simulink model "dart_AUV_simulink_model"  (R2024b)
settings: Solver=VariableStepAuto  StartTime=0.0  StopTime=20  RelTol=1e-3
values from neighbouring files (symbols this model uses):
  Af = [0.5; 0.1; 0.5]    [init_param.m]
  Bc = [0, 0, 0.042]    [init_param.m]
  Cg = [0, 0, 0.021]    [init_param.m]
  Delta_2 = Delta.^2    [init_param.m]
  DL = diag([Xu, 0, 0, 0, 0, 0 ... (first row only)    [init_param.m]
  DNL = diag([Xu_nl, 0, 0, 0, 0, 0 ... (first row only)    [init_param.m]
  I = [Ixx,Iyy, Izz, Ixy, Ixz, Iyz]    [init_param.m]
  L = 0.47    [init_param.m]
  m = 2.24    [init_param.m]
  Ma = [ ... (first row only)    [init_param.m]
  Mt = Mb + Ma    [init_param.m]
  Omega = [0.085; 0.085; 0.9]    [init_param.m]
  R = d / 2    (= 0.04445)    [init_param.m]
  rho = 1025    [init_param.m]
undefined symbols (not defined in the file or in its folder): CD, CL, fractalcoef
libraries: slpidlib x3, mspfiltlib x1, mspsensorlib x1, mpclib x1
settings Model: Creator=tihan  LastModifiedBy=tihan

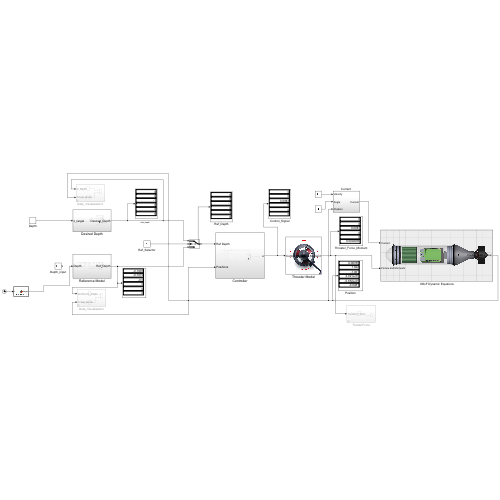
[thumbnail: Simulink's stored preview of the top-level diagram]
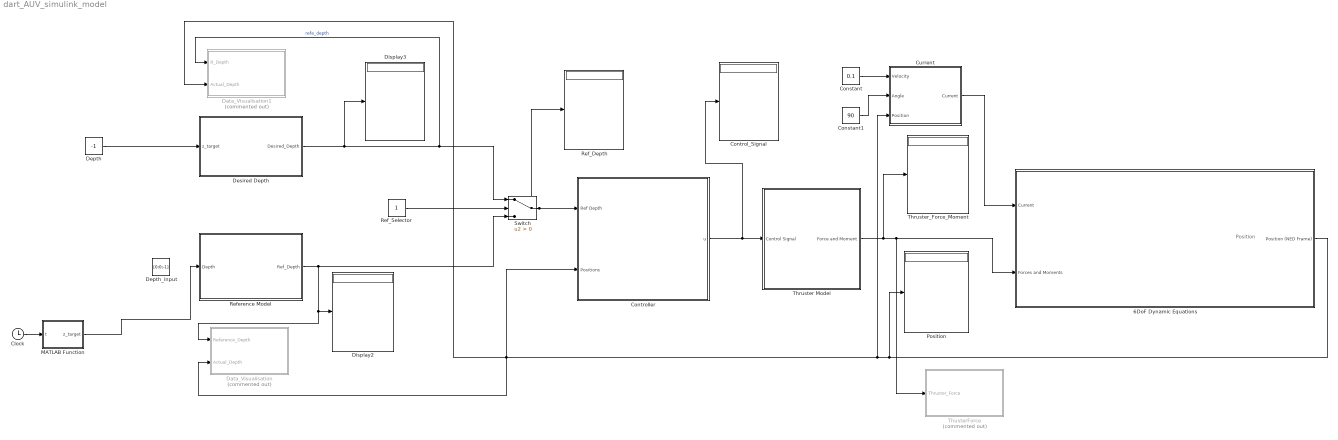
== system dart_AUV_simulink_model ==
  note: Position
  " 6DoF Dynamic Equations " : Subsystem
      mask Display: image('image.png');
  Clock : Clock
  Constant : Constant  Value=0.1
  Constant1 : Constant  Value=90
  Control_Signal : Display
  Controller : Subsystem
  "Current " : Subsystem
  Data_Visualisation : Subsystem  Commented=on
  Data_Visualisation1 : Subsystem  Commented=on
  Depth : Constant  Value=-1
  Depth_input : Constant  Value=[0;0;-1]
  Desired Depth : Subsystem
  Display2 : Display
  Display3 : Display
  MATLAB Function : MATLAB Function  TreatAsAtomicUnit=on
  Position : Display
  Ref_Depth : Display
  Ref_Selector : Constant
  Reference Model : Subsystem
  Switch : Switch  Criteria=u2 > Threshold  SaturateOnIntegerOverflow=off  InputSameDT=off
  Thruster Model : Subsystem
      mask Display: image('thruster_small.jpg');
  Thruster_Force_Moment : Display
  ThusterForce : Subsystem  Commented=on
  wires:
  Controller/1(u) -> Thruster Model/1(Control Signal), Control_Signal/1
  " 6DoF Dynamic Equations "/1(Position (NED Frame)) -> Position/1, Controller/2(Positions), Data_Visualisation1/2(Actual_Depth), Data_Visualisation/2(Actual_Depth), "Current "/3(Position)
  Thruster Model/1(Force and Moment) -> ThusterForce/1(Thruster_Force), " 6DoF Dynamic Equations "/2("Forces and Moments  "), Thruster_Force_Moment/1
  Reference Model/1(Ref_Depth) -> Switch/3, Data_Visualisation/1(Reference_Depth), Display2/1
  "Current "/1(Current) -> " 6DoF Dynamic Equations "/1(Current)
  Constant/1 -> "Current "/1(Velocity)
  Constant1/1 -> "Current "/2(Angle)
  Ref_Selector/1 -> Switch/2
  Switch/1 -> Controller/1(Ref Depth), Ref_Depth/1
  Desired Depth/1(Desired_Depth) -> Display3/1, Data_Visualisation1/1(R_Depth), Switch/1  "refe_depth"
  Clock/1 -> MATLAB Function/1(t)
  MATLAB Function/1(z_target) -> Reference Model/1(Depth)
  Depth/1 -> Desired Depth/1(z_target)

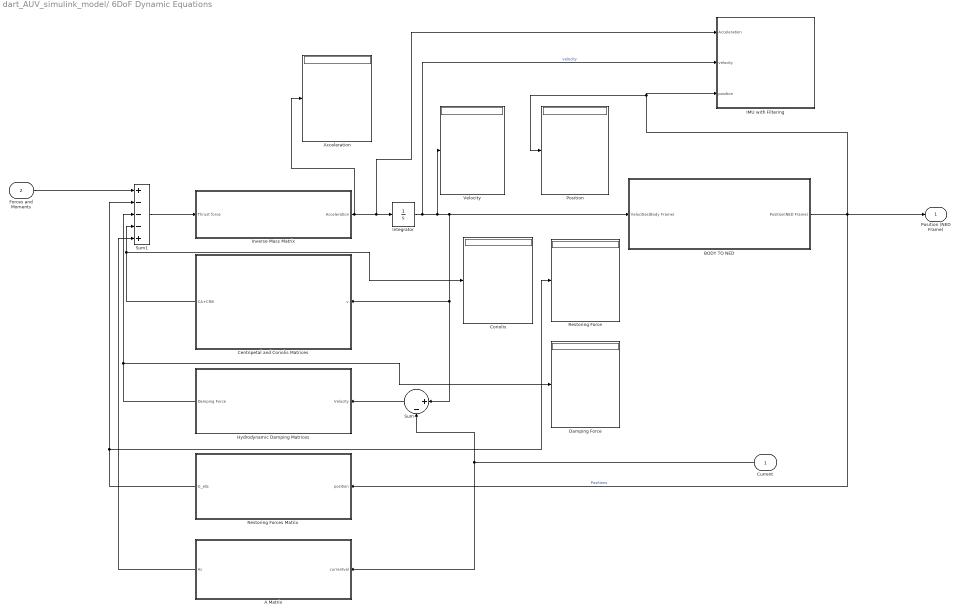
== system dart_AUV_simulink_model/ 6DoF Dynamic Equations  ==
  Current : Inport
  "Forces and Moments  " : Inport  Port=2
  " A Matrix" : Subsystem
  Acceleration : Display
  BODY TO NED : Subsystem
  "Centripetal and Coriolis Matrices " : Subsystem
  Coriolis : Display
  Damping Force : Display
  "Hydrodynamic Damping Matrices " : Subsystem
  IMU with Filtering : Subsystem
  Integrator : Integrator
  Inverse Mass Matrix : Subsystem
  Position : Display
  Restoring Force : Display
  Restoring Forces Matrix : Subsystem
  Sum : Sum  Inputs=|+-
  Sum1 : Sum  Inputs=+---+  InputSameDT=on  SaturateOnIntegerOverflow=on  OutDataTypeStr=Inherit: Same as first input
  Velocity : Display
  Position (NED Frame) : Outport  VectorParamsAs1DForOutWhenUnconnected=off
  wires:
  Restoring Forces Matrix/1(G_eta) -> Restoring Force/1, Sum1/2
  Sum1/1 -> Inverse Mass Matrix/1(Thrust force)
  "Forces and Moments  "/1 -> Sum1/1
  "Centripetal and Coriolis Matrices "/1(CA+CRB) -> Coriolis/1, Sum1/4
  Sum/1 -> "Hydrodynamic Damping Matrices "/1(Velocity)
  Current/1 -> " A Matrix"/1(currentvel), Sum/2
  " A Matrix"/1(Ac) -> Sum1/5
  Inverse Mass Matrix/1(Acceleration) -> IMU with Filtering/1(Acceleration), Integrator/1, Acceleration/1
  Integrator/1 -> IMU with Filtering/2(velocity), Velocity/1, "Centripetal and Coriolis Matrices "/1(v), Sum/1, BODY TO NED/1(Velocities(Body Frame))  "velocity"
  "Hydrodynamic Damping Matrices "/1(Damping Force) -> Damping Force/1, Sum1/3
  BODY TO NED/1(" Position(NED Frame)") -> Restoring Forces Matrix/1(position), IMU with Filtering/3(position), Position/1, Position (NED Frame)/1  "Positions"

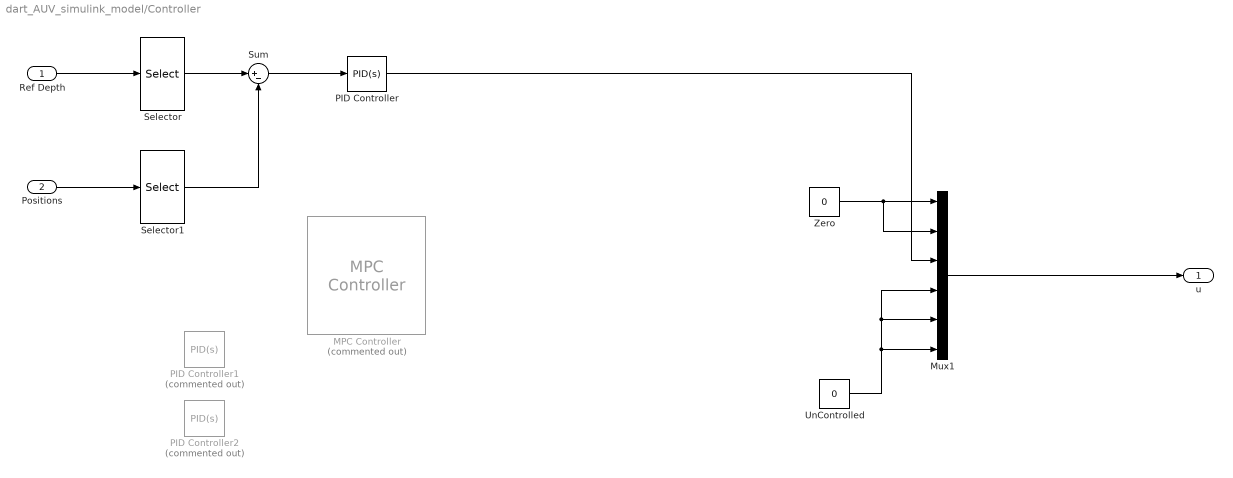
== system dart_AUV_simulink_model/Controller ==
  Ref Depth : Inport
  Positions : Inport  Port=2
  MPC Controller : mpclib/MPC Controller  Commented=on  SCDEnableBlockLinearizationSpecification=on  is_multiple=0  enable_value=0  return_u0=off  updateMPCinCallerWorkspace=on  md_inport=off  mv_inport=off  uref_inport=off  return_cost=off  return_mvseq=off  return_qpstatus=off  return_xseq=off  return_state=off  return_ovseq=off  state_inport=off  umin_inport=off  umax_inport=off  ymin_inport=off  ymax_inport=off  cc_inport=off  ywt_inport=off  uwt_inport=off  duwt_inport=off  rhoeps_inport=off  pm_inport=off  MaximumP=10  HorizonChoice=FixedHorizon  n_ts=1  n_p=10  n_mv=1  n_md=1  n_ud=0  n_mo=1  n_uo=0  BlockDataType=double  SampleTimeInherited=off  switch_inport=off
  Mux1 : Mux  Inputs=6
  PID Controller : slpidlib/PID Controller  Controller=PID  Form=Parallel  TimeDomain=Continuous-time  UseExternalTs=off  SampleTime=-1  IntegratorMethod=Forward Euler  FilterMethod=Forward Euler  ControllerParametersSource=internal  P=80  I=0.001  UseKiTs=off  D=50  UseExternalDerivativeSource=off  N=114.923982318212  UseFilter=on  TunerSelectOption=Transfer Function Based (PID Tuner App)  InitialConditionSource=internal  InitialConditionForIntegrator=0  InitialConditionForFilter=0  DifferentiatorICPrevScaledInput=0  ExternalReset=none  TrackingMode=off  Kt=1  LimitOutput=off  SatLimitsSource=internal  UpperSaturationLimit=inf  LowerSaturationLimit=-inf  LinearizeAsGain=on  AntiWindupMode=none  Kb=1  LimitIntegrator=off  UpperIntegratorSaturationLimit=inf  LowerIntegratorSaturationLimit=-inf  POutMin=[]  POutMax=[]  IOutMin=[]  IOutMax=[]  DOutMin=[]  DOutMax=[]  NOutMin=[]  NOutMax=[]  SumOutMin=[]  SumOutMax=[]  SaturationOutMin=[]  SaturationOutMax=[]  PParamMin=[]  PParamMax=[]  IParamMin=[]  IParamMax=[]  DParamMin=[]  DParamMax=[]  NParamMin=[]  NParamMax=[]  KbParamMin=[]  KbParamMax=[]  KtParamMin=[]  KtParamMax=[]  KbOutMin=[]  KbOutMax=[]  KtOutMin=[]  KtOutMax=[]  IntegratorOutMin=[]  IntegratorOutMax=[]  FilterOutMin=[]  FilterOutMax=[]  SumI1OutMin=[]  SumI1OutMax=[]  SumI2OutMin=[]  SumI2OutMax=[]  SumI3OutMin=[]  SumI3OutMax=[]  SumI4OutMin=[]  SumI4OutMax=[]  SumDOutMin=[]  SumDOutMax=[]  DifferentiatorOutMin=[]  DifferentiatorOutMax=[]  FilterDiffOutCoefMin=[]  FilterDiffOutCoefMax=[]  ReciprocalOutMin=[]  ReciprocalOutMax=[]  SumDenOutMin=[]  SumDenOutMax=[]  SumNumOutMin=[]  SumNumOutMax=[]  DivideOutMin=[]  DivideOutMax=[]  UdiffTsProdOutMin=[]  UdiffTsProdOutMax=[]  NTsProdOutMin=[]  NTsProdOutMax=[]  UintegralTsProdOutMin=[]  UintegralTsProdOutMax=[]  UngainTsProdOutMin=[]  UngainTsProdOutMax=[]  ClampingZeroOutDataTypeStr=Inherit: Inherit via back propagation  ClampingZeroOutMin=[]  ClampingZeroOutMax=[]  FilterDenConstantOutDataTypeStr=Inherit: Inherit via back propagation  FilterDenConstantOutMin=[]  FilterDenConstantOutMax=[]  PCopyOutDataTypeStr=Inherit: Inherit via back propagation  PCopyOutMin=[]  PCopyOutMax=[]  NCopyOutDataTypeStr=Inherit: Inherit via back propagation  NCopyOutMin=[]  NCopyOutMax=[]  IntegratorContinuousStateAttributes=''  IntegratorStateMustResolveToSignalObject=off  IntegratorRTWStateStorageClass=Auto  FilterContinuousStateAttributes=''  FilterStateMustResolveToSignalObject=off  FilterRTWStateStorageClass=Auto  ParallelPVariant=InternalParameters  IdealPVariant=Disabled  IVariant=InternalParameters  DVariant=InternalParameters  IntegratorVariant=Continuous  SatVariant=Disabled  AWVariant=Passthrough  PCopyVariant=Disabled  TRVariant=Disabled  FdbkBlocksVariant=Forward  IdealPFdbkVariant=Disabled  SatFdbkVariant=Disabled  DerivativeFilterVariant=ContFilter  NVariant=InternalParameters  NCopyVariant=Disabled  FilterICVariant=InternalICsFilter  IntegratorICVariant=InternalICs  ExternalResetVariant=Disabled  TRSumVariant=Passthrough  SumFdbkVariant=Disabled  SumVariant=Sum_PID  TsampFilterVariant=InternalTs  TsampNgainVariant=Passthrough  TsampIntegralVariant=Disabled_SignalSpec  ExternalSaturationOutDataTypeStr=Inherit: Same as second input  DerivativeSourceVariant=ErrorSignal  PreIntVariant=InternalPreInt
  PID Controller1 : slpidlib/PID Controller  Commented=on  Controller=PID  Form=Parallel  TimeDomain=Continuous-time  UseExternalTs=off  SampleTime=-1  IntegratorMethod=Forward Euler  FilterMethod=Forward Euler  ControllerParametersSource=internal  P=90  I=0.1  UseKiTs=off  D=70  UseExternalDerivativeSource=off  N=257.686519224459  UseFilter=on  TunerSelectOption=Transfer Function Based (PID Tuner App)  InitialConditionSource=internal  InitialConditionForIntegrator=0  InitialConditionForFilter=0  DifferentiatorICPrevScaledInput=0  ExternalReset=none  TrackingMode=off  Kt=1  LimitOutput=off  SatLimitsSource=internal  UpperSaturationLimit=inf  LowerSaturationLimit=-inf  LinearizeAsGain=on  AntiWindupMode=none  Kb=1  LimitIntegrator=off  UpperIntegratorSaturationLimit=inf  LowerIntegratorSaturationLimit=-inf  POutMin=[]  POutMax=[]  IOutMin=[]  IOutMax=[]  DOutMin=[]  DOutMax=[]  NOutMin=[]  NOutMax=[]  SumOutMin=[]  SumOutMax=[]  SaturationOutMin=[]  SaturationOutMax=[]  PParamMin=[]  PParamMax=[]  IParamMin=[]  IParamMax=[]  DParamMin=[]  DParamMax=[]  NParamMin=[]  NParamMax=[]  KbParamMin=[]  KbParamMax=[]  KtParamMin=[]  KtParamMax=[]  KbOutMin=[]  KbOutMax=[]  KtOutMin=[]  KtOutMax=[]  IntegratorOutMin=[]  IntegratorOutMax=[]  FilterOutMin=[]  FilterOutMax=[]  SumI1OutMin=[]  SumI1OutMax=[]  SumI2OutMin=[]  SumI2OutMax=[]  SumI3OutMin=[]  SumI3OutMax=[]  SumI4OutMin=[]  SumI4OutMax=[]  SumDOutMin=[]  SumDOutMax=[]  DifferentiatorOutMin=[]  DifferentiatorOutMax=[]  FilterDiffOutCoefMin=[]  FilterDiffOutCoefMax=[]  ReciprocalOutMin=[]  ReciprocalOutMax=[]  SumDenOutMin=[]  SumDenOutMax=[]  SumNumOutMin=[]  SumNumOutMax=[]  DivideOutMin=[]  DivideOutMax=[]  UdiffTsProdOutMin=[]  UdiffTsProdOutMax=[]  NTsProdOutMin=[]  NTsProdOutMax=[]  UintegralTsProdOutMin=[]  UintegralTsProdOutMax=[]  UngainTsProdOutMin=[]  UngainTsProdOutMax=[]  ClampingZeroOutDataTypeStr=Inherit: Inherit via back propagation  ClampingZeroOutMin=[]  ClampingZeroOutMax=[]  FilterDenConstantOutDataTypeStr=Inherit: Inherit via back propagation  FilterDenConstantOutMin=[]  FilterDenConstantOutMax=[]  PCopyOutDataTypeStr=Inherit: Inherit via back propagation  PCopyOutMin=[]  PCopyOutMax=[]  NCopyOutDataTypeStr=Inherit: Inherit via back propagation  NCopyOutMin=[]  NCopyOutMax=[]  IntegratorContinuousStateAttributes=''  IntegratorStateMustResolveToSignalObject=off  IntegratorRTWStateStorageClass=Auto  FilterContinuousStateAttributes=''  FilterStateMustResolveToSignalObject=off  FilterRTWStateStorageClass=Auto  ParallelPVariant=InternalParameters  IdealPVariant=Disabled  IVariant=InternalParameters  DVariant=InternalParameters  IntegratorVariant=Continuous  SatVariant=Disabled  AWVariant=Passthrough  PCopyVariant=Disabled  TRVariant=Disabled  FdbkBlocksVariant=Forward  IdealPFdbkVariant=Disabled  SatFdbkVariant=Disabled  DerivativeFilterVariant=ContFilter  NVariant=InternalParameters  NCopyVariant=Disabled  FilterICVariant=InternalICsFilter  IntegratorICVariant=InternalICs  ExternalResetVariant=Disabled  TRSumVariant=Passthrough  SumFdbkVariant=Disabled  SumVariant=Sum_PID  TsampFilterVariant=InternalTs  TsampNgainVariant=Passthrough  TsampIntegralVariant=Disabled_SignalSpec  ExternalSaturationOutDataTypeStr=Inherit: Same as second input  DerivativeSourceVariant=ErrorSignal  PreIntVariant=InternalPreInt
  PID Controller2 : slpidlib/PID Controller  Commented=on  Controller=PID  Form=Parallel  TimeDomain=Continuous-time  UseExternalTs=off  SampleTime=-1  IntegratorMethod=Forward Euler  FilterMethod=Forward Euler  ControllerParametersSource=internal  P=90  I=.1  UseKiTs=off  D=70  UseExternalDerivativeSource=off  N=257.686519224459  UseFilter=on  TunerSelectOption=Transfer Function Based (PID Tuner App)  InitialConditionSource=internal  InitialConditionForIntegrator=0  InitialConditionForFilter=0  DifferentiatorICPrevScaledInput=0  ExternalReset=none  TrackingMode=off  Kt=1  LimitOutput=off  SatLimitsSource=internal  UpperSaturationLimit=inf  LowerSaturationLimit=-inf  LinearizeAsGain=on  AntiWindupMode=none  Kb=1  LimitIntegrator=off  UpperIntegratorSaturationLimit=inf  LowerIntegratorSaturationLimit=-inf  POutMin=[]  POutMax=[]  IOutMin=[]  IOutMax=[]  DOutMin=[]  DOutMax=[]  NOutMin=[]  NOutMax=[]  SumOutMin=[]  SumOutMax=[]  SaturationOutMin=[]  SaturationOutMax=[]  PParamMin=[]  PParamMax=[]  IParamMin=[]  IParamMax=[]  DParamMin=[]  DParamMax=[]  NParamMin=[]  NParamMax=[]  KbParamMin=[]  KbParamMax=[]  KtParamMin=[]  KtParamMax=[]  KbOutMin=[]  KbOutMax=[]  KtOutMin=[]  KtOutMax=[]  IntegratorOutMin=[]  IntegratorOutMax=[]  FilterOutMin=[]  FilterOutMax=[]  SumI1OutMin=[]  SumI1OutMax=[]  SumI2OutMin=[]  SumI2OutMax=[]  SumI3OutMin=[]  SumI3OutMax=[]  SumI4OutMin=[]  SumI4OutMax=[]  SumDOutMin=[]  SumDOutMax=[]  DifferentiatorOutMin=[]  DifferentiatorOutMax=[]  FilterDiffOutCoefMin=[]  FilterDiffOutCoefMax=[]  ReciprocalOutMin=[]  ReciprocalOutMax=[]  SumDenOutMin=[]  SumDenOutMax=[]  SumNumOutMin=[]  SumNumOutMax=[]  DivideOutMin=[]  DivideOutMax=[]  UdiffTsProdOutMin=[]  UdiffTsProdOutMax=[]  NTsProdOutMin=[]  NTsProdOutMax=[]  UintegralTsProdOutMin=[]  UintegralTsProdOutMax=[]  UngainTsProdOutMin=[]  UngainTsProdOutMax=[]  ClampingZeroOutDataTypeStr=Inherit: Inherit via back propagation  ClampingZeroOutMin=[]  ClampingZeroOutMax=[]  FilterDenConstantOutDataTypeStr=Inherit: Inherit via back propagation  FilterDenConstantOutMin=[]  FilterDenConstantOutMax=[]  PCopyOutDataTypeStr=Inherit: Inherit via back propagation  PCopyOutMin=[]  PCopyOutMax=[]  NCopyOutDataTypeStr=Inherit: Inherit via back propagation  NCopyOutMin=[]  NCopyOutMax=[]  IntegratorContinuousStateAttributes=''  IntegratorStateMustResolveToSignalObject=off  IntegratorRTWStateStorageClass=Auto  FilterContinuousStateAttributes=''  FilterStateMustResolveToSignalObject=off  FilterRTWStateStorageClass=Auto  ParallelPVariant=InternalParameters  IdealPVariant=Disabled  IVariant=InternalParameters  DVariant=InternalParameters  IntegratorVariant=Continuous  SatVariant=Disabled  AWVariant=Passthrough  PCopyVariant=Disabled  TRVariant=Disabled  FdbkBlocksVariant=Forward  IdealPFdbkVariant=Disabled  SatFdbkVariant=Disabled  DerivativeFilterVariant=ContFilter  NVariant=InternalParameters  NCopyVariant=Disabled  FilterICVariant=InternalICsFilter  IntegratorICVariant=InternalICs  ExternalResetVariant=Disabled  TRSumVariant=Passthrough  SumFdbkVariant=Disabled  SumVariant=Sum_PID  TsampFilterVariant=InternalTs  TsampNgainVariant=Passthrough  TsampIntegralVariant=Disabled_SignalSpec  ExternalSaturationOutDataTypeStr=Inherit: Same as second input  DerivativeSourceVariant=ErrorSignal  PreIntVariant=InternalPreInt
  Selector : Selector  InputPortWidth=6  IndexOptions=Index vector (dialog)  Indices=[3]  OutputSizes=1
  Selector1 : Selector  InputPortWidth=6  IndexOptions=Index vector (dialog)  Indices=[3]  OutputSizes=1
  Sum : Sum  Inputs=|+-
  UnControlled : Constant  Value=0
  Zero : Constant  Value=0
  u : Outport
  wires:
  Ref Depth/1 -> Selector/1
  Positions/1 -> Selector1/1
  Selector/1 -> Sum/1
  Selector1/1 -> Sum/2
  Sum/1 -> PID Controller/1
  Zero/1 -> Mux1/2, Mux1/1
  Mux1/1 -> u/1
  UnControlled/1 -> Mux1/4, Mux1/5, Mux1/6
  PID Controller/1 -> Mux1/3

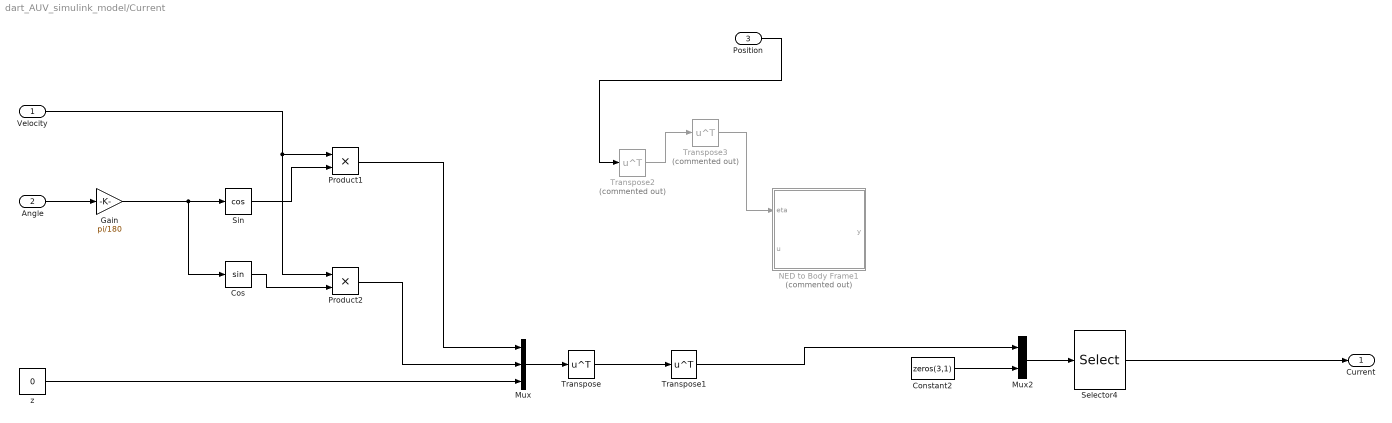
== system dart_AUV_simulink_model/Current  ==
  Velocity : Inport
  Angle : Inport  Port=2
  Position : Inport  Port=3
  Constant2 : Constant  Value=zeros(3,1)
  Cos : Trigonometry
  Gain : Gain  Gain=pi/180
  Mux : Mux  Inputs=3
  Mux2 : Mux  Inputs=2
  NED to Body Frame1 : MATLAB Function  Commented=on  TreatAsAtomicUnit=on
  Product1 : Product
  Product2 : Product
  Selector4 : Selector  InputPortWidth=6  IndexOptions=Index vector (dialog)  Indices=[1 2 4 5 6 3]  OutputSizes=1
  Sin : Trigonometry  Operator=cos  OutputSignalType=real
  Transpose : Math  Operator=transpose
  Transpose1 : Math  Operator=transpose
  Transpose2 : Math  Commented=on  Operator=transpose
  Transpose3 : Math  Commented=on  Operator=transpose
  z : Constant  Value=0
  Current : Outport  VectorParamsAs1DForOutWhenUnconnected=off
  wires:
  Selector4/1 -> Current/1
  Mux2/1 -> Selector4/1
  Mux/1 -> Transpose/1
  Velocity/1 -> Product2/1, Product1/1
  Sin/1 -> Product1/2
  Cos/1 -> Product2/2
  Product1/1 -> Mux/1
  Product2/1 -> Mux/2
  z/1 -> Mux/3
  Transpose/1 -> Transpose1/1
  Angle/1 -> Gain/1
  Constant2/1 -> Mux2/2
  Gain/1 -> Cos/1, Sin/1
  Transpose2/1 -> Transpose3/1
  Transpose3/1 -> NED to Body Frame1/1(eta)
  Position/1 -> Transpose2/1
  Transpose1/1 -> Mux2/1

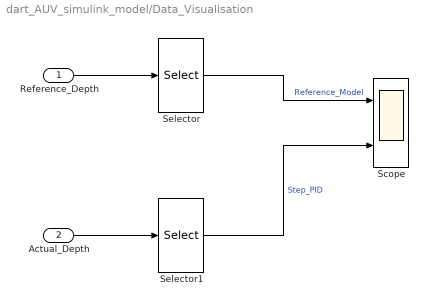
== system dart_AUV_simulink_model/Data_Visualisation ==
  Reference_Depth : Inport
  Actual_Depth : Inport  Port=2
  Scope : Scope  NumInputPorts=2
  Selector : Selector  InputPortWidth=6  IndexOptions=Index vector (dialog)  Indices=[3]  OutputSizes=1
  Selector1 : Selector  InputPortWidth=6  IndexOptions=Index vector (dialog)  Indices=[3]  OutputSizes=1
  wires:
  Reference_Depth/1 -> Selector/1
  Actual_Depth/1 -> Selector1/1
  Selector/1 -> Scope/1  "Reference_Model"
  Selector1/1 -> Scope/2  "Step_PID"

== system dart_AUV_simulink_model/Data_Visualisation1 ==
  R_Depth : Inport
  Actual_Depth : Inport  Port=2
  Scope : Scope  NumInputPorts=2
  Selector : Selector  InputPortWidth=6  IndexOptions=Index vector (dialog)  Indices=[3]  OutputSizes=1
  Selector1 : Selector  InputPortWidth=6  IndexOptions=Index vector (dialog)  Indices=[3]  OutputSizes=1
  wires:
  Selector1/1 -> Scope/2  "Actual_Depth"
  Selector/1 -> Scope/1  "R_Depth"
  Actual_Depth/1 -> Selector1/1
  R_Depth/1 -> Selector/1

== system dart_AUV_simulink_model/Desired Depth ==
  z_target : Inport
  Mux1 : Mux  Inputs=6
  UnControlled : Constant  Value=0
  Zero : Constant  Value=0
  Desired_Depth : Outport
  wires:
  UnControlled/1 -> Mux1/4, Mux1/5, Mux1/6
  Zero/1 -> Mux1/2, Mux1/1
  Mux1/1 -> Desired_Depth/1
  z_target/1 -> Mux1/3

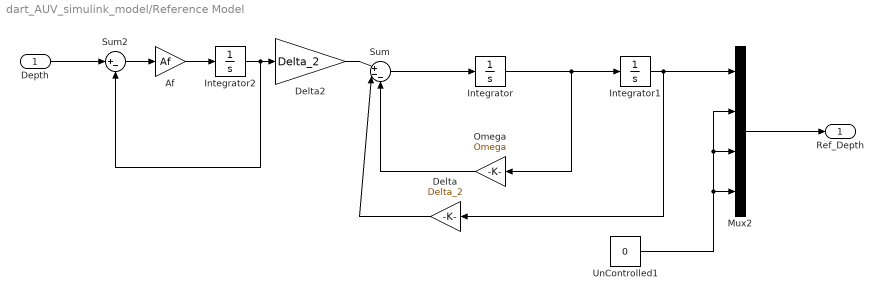
== system dart_AUV_simulink_model/Reference Model ==
  Depth : Inport
  Af : Gain  Gain=Af
  Delta : Gain  Gain=Delta_2
  Delta2 : Gain  Gain=Delta_2
  Integrator : Integrator
  Integrator1 : Integrator
  Integrator2 : Integrator
  Mux2 : Mux
  Omega : Gain  Gain=Omega
  Sum : Sum  Inputs=|+--
  Sum2 : Sum  Inputs=|+-
  UnControlled1 : Constant  Value=0
  Ref_Depth : Outport
  wires:
  Depth/1 -> Sum2/1
  Omega/1 -> Sum/3
  Sum2/1 -> Af/1
  Delta/1 -> Sum/2
  Af/1 -> Integrator2/1
  Integrator1/1 -> Mux2/1, Delta/1
  Integrator/1 -> Integrator1/1, Omega/1
  Integrator2/1 -> Delta2/1, Sum2/2
  Delta2/1 -> Sum/1
  Sum/1 -> Integrator/1
  UnControlled1/1 -> Mux2/2, Mux2/3, Mux2/4
  Mux2/1 -> Ref_Depth/1

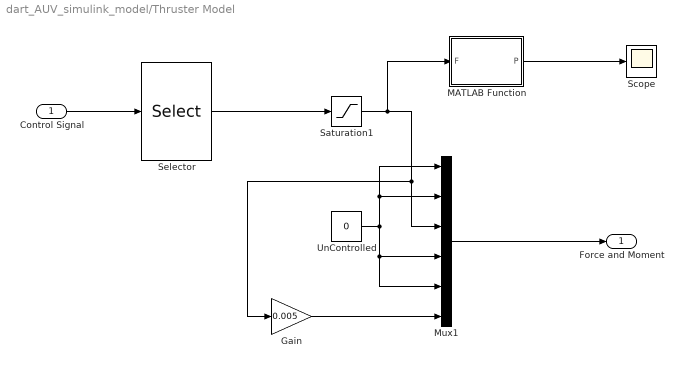
== system dart_AUV_simulink_model/Thruster Model ==
  Control Signal : Inport
  Gain : Gain  Gain=0.005
  MATLAB Function : MATLAB Function  TreatAsAtomicUnit=on
  Mux1 : Mux  Inputs=6
  Saturation1 : Saturate  UpperLimit=1.7  LowerLimit=-1.6
  Scope : Scope
  Selector : Selector  InputPortWidth=6  IndexOptions=Index vector (dialog)  Indices=[3]  OutputSizes=1
  UnControlled : Constant  Value=0
  Force and Moment : Outport
  wires:
  UnControlled/1 -> Mux1/4, Mux1/5, Mux1/1, Mux1/2
  Control Signal/1 -> Selector/1
  Mux1/1 -> Force and Moment/1
  Selector/1 -> Saturation1/1
  Gain/1 -> Mux1/6
  Saturation1/1 -> MATLAB Function/1(F), Gain/1, Mux1/3
  MATLAB Function/1(P) -> Scope/1

== system dart_AUV_simulink_model/ThusterForce ==
  Thruster_Force : Inport
  Scope : Scope
  Selector : Selector  InputPortWidth=6  IndexOptions=Index vector (dialog)  Indices=[3]  OutputSizes=1
  wires:
  Selector/1 -> Scope/1  "Thruster_Froce"
  Thruster_Force/1 -> Selector/1

== system dart_AUV_simulink_model/ 6DoF Dynamic Equations / A Matrix ==
  currentvel : Inport
  MA : Gain  Gain=Ma  Multiplication=Matrix(K*u)  OutDataTypeStr=Inherit: Same as input  ParamDataTypeStr=Inherit: Same as input
  MATLAB Function : MATLAB Function  TreatAsAtomicUnit=on
  Ac : Outport
  wires:
  MATLAB Function/1(y) -> MA/1
  MA/1 -> Ac/1
  currentvel/1 -> MATLAB Function/1(data), MATLAB Function/2(u)

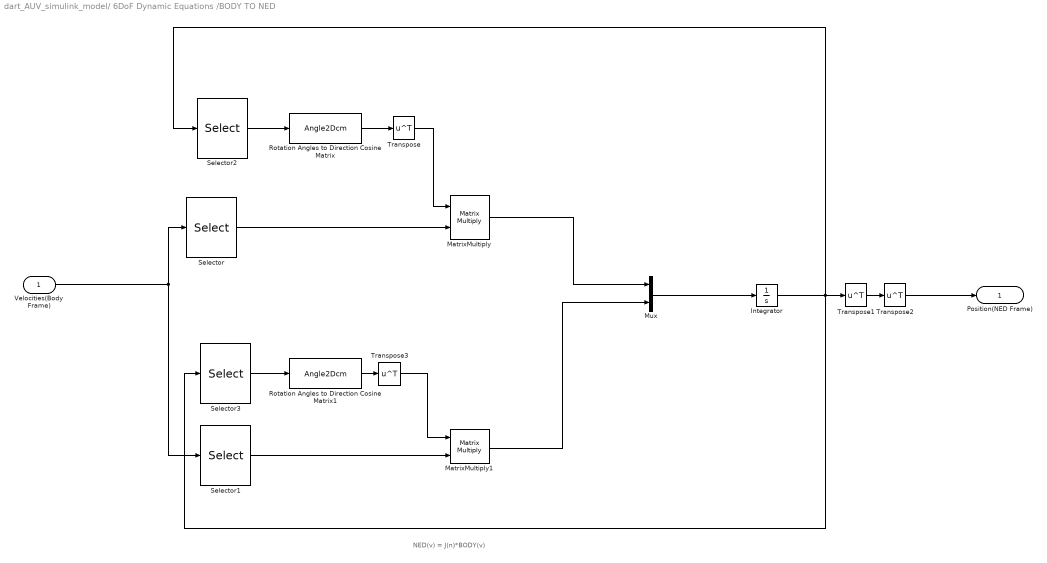
== system dart_AUV_simulink_model/ 6DoF Dynamic Equations /BODY TO NED ==
  note: NED(v) = J(n)*BODY(v)
  Velocities(Body Frame) : Inport
  Integrator : Integrator
  MatrixMultiply : Product  Multiplication=Matrix(*)
  MatrixMultiply1 : Product  Multiplication=Matrix(*)
  Mux : Mux  Inputs=2
  Rotation Angles to Direction Cosine Matrix : Angle2Dcm  rotationOrder=XYZ
      settings: AttributesFormatString=Rotation Order: %<rotationOrder>
  Rotation Angles to Direction Cosine Matrix1 : Angle2Dcm  rotationOrder=XYZ
      settings: AttributesFormatString=Rotation Order: %<rotationOrder>
  Selector : Selector  InputPortWidth=6  IndexOptions=Index vector (dialog)  Indices=[1 2 3]  OutputSizes=1
  Selector1 : Selector  InputPortWidth=6  IndexOptions=Index vector (dialog)  Indices=[ 4 5 6]  OutputSizes=1
  Selector2 : Selector  InputPortWidth=6  IndexOptions=Index vector (dialog)  Indices=[ 4 5 6]  OutputSizes=1
  Selector3 : Selector  InputPortWidth=6  IndexOptions=Index vector (dialog)  Indices=[ 4 5 6]  OutputSizes=1
  Transpose{,1..3} (4 alike) : Math  Operator=transpose
  " Position(NED Frame)" : Outport
  wires:
  Velocities(Body Frame)/1 -> Selector/1, Selector1/1
  Selector/1 -> MatrixMultiply/2
  Selector1/1 -> MatrixMultiply1/2
  MatrixMultiply/1 -> Mux/1
  MatrixMultiply1/1 -> Mux/2
  Mux/1 -> Integrator/1
  Integrator/1 -> Selector2/1, Transpose1/1, Selector3/1
  Selector2/1 -> Rotation Angles to Direction Cosine Matrix/1
  Rotation Angles to Direction Cosine Matrix/1 -> Transpose/1
  Transpose/1 -> MatrixMultiply/1
  Transpose1/1 -> Transpose2/1
  Transpose2/1 -> " Position(NED Frame)"/1
  Selector3/1 -> Rotation Angles to Direction Cosine Matrix1/1
  Rotation Angles to Direction Cosine Matrix1/1 -> Transpose3/1
  Transpose3/1 -> MatrixMultiply1/1

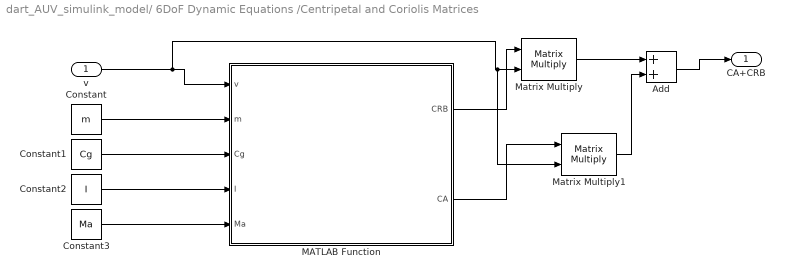
== system dart_AUV_simulink_model/ 6DoF Dynamic Equations /Centripetal and Coriolis Matrices  ==
  v : Inport
  Add : Sum
  Constant : Constant  Value=m
  Constant1 : Constant  Value=Cg
  Constant2 : Constant  Value=I
  Constant3 : Constant  Value=Ma
  MATLAB Function : MATLAB Function  TreatAsAtomicUnit=on
  Matrix Multiply : Product  Multiplication=Matrix(*)
  Matrix Multiply1 : Product  Multiplication=Matrix(*)
  CA+CRB : Outport
  wires:
  Constant/1 -> MATLAB Function/2(m)
  Constant1/1 -> MATLAB Function/3(Cg)
  Constant2/1 -> MATLAB Function/4(I)
  Constant3/1 -> MATLAB Function/5(Ma)
  v/1 -> Matrix Multiply1/2, Matrix Multiply/2, MATLAB Function/1(v)
  MATLAB Function/2(CA) -> Matrix Multiply1/1
  MATLAB Function/1(CRB) -> Matrix Multiply/1
  Matrix Multiply/1 -> Add/1
  Matrix Multiply1/1 -> Add/2
  Add/1 -> CA+CRB/1

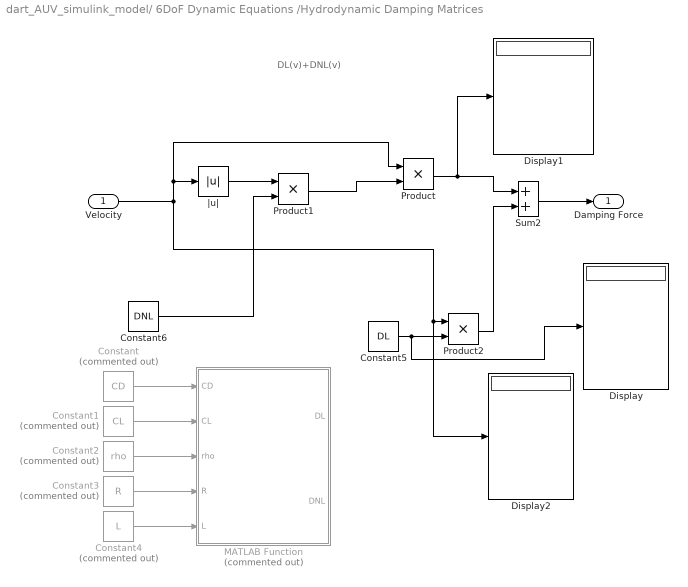
== system dart_AUV_simulink_model/ 6DoF Dynamic Equations /Hydrodynamic Damping Matrices  ==
  note: DL(v)+DNL(v)
  Velocity : Inport
  Constant : Constant  Commented=on  Value=CD
  Constant1 : Constant  Commented=on  Value=CL
  Constant2 : Constant  Commented=on  Value=rho
  Constant3 : Constant  Commented=on  Value=R
  Constant4 : Constant  Commented=on  Value=L
  Constant5 : Constant  Value=DL
  Constant6 : Constant  Value=DNL
  Display : Display
  Display1 : Display
  Display2 : Display
  MATLAB Function : MATLAB Function  Commented=on  TreatAsAtomicUnit=on
  Product : Product  InputSameDT=on  RndMeth=Zero  SaturateOnIntegerOverflow=on  OutDataTypeStr=Inherit: Same as first input
  Product1 : Product  InputSameDT=on  RndMeth=Zero  SaturateOnIntegerOverflow=on  OutDataTypeStr=Inherit: Same as first input
  Product2 : Product  InputSameDT=on  RndMeth=Zero  SaturateOnIntegerOverflow=on  OutDataTypeStr=Inherit: Same as first input
  Sum2 : Sum  InputSameDT=on  SaturateOnIntegerOverflow=on  OutDataTypeStr=Inherit: Same as first input
  |u| : Abs
  Damping Force : Outport
  wires:
  Product/1 -> Display1/1, Sum2/1
  |u|/1 -> Product1/1
  Sum2/1 -> Damping Force/1
  Velocity/1 -> Display2/1, Product2/1, Product/1, |u|/1
  Constant4/1 -> MATLAB Function/5(L)
  Constant3/1 -> MATLAB Function/4(R)
  Constant2/1 -> MATLAB Function/3(rho)
  Constant1/1 -> MATLAB Function/2(CL)
  Constant/1 -> MATLAB Function/1(CD)
  Product2/1 -> Sum2/2
  Product1/1 -> Product/2
  Constant5/1 -> Display/1, Product2/2
  Constant6/1 -> Product1/2

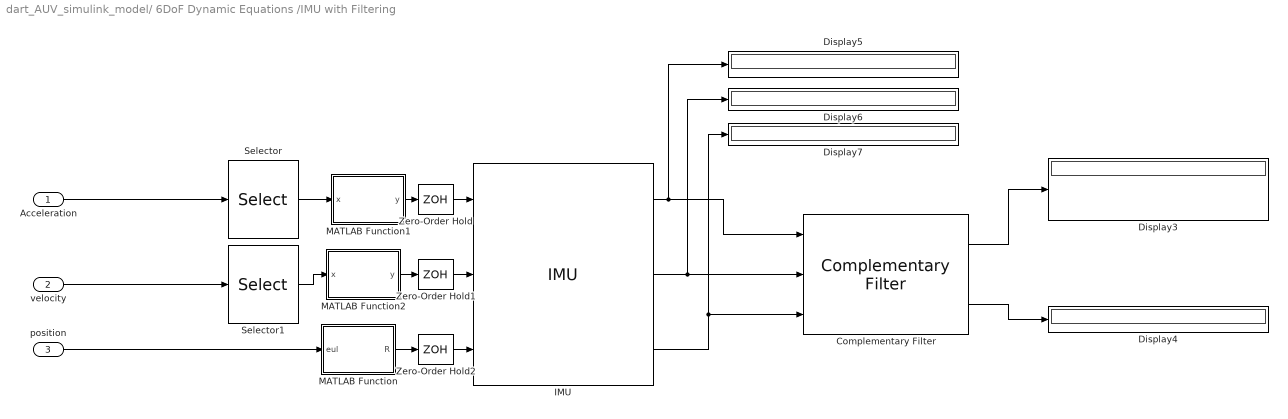
== system dart_AUV_simulink_model/ 6DoF Dynamic Equations /IMU with Filtering ==
  Acceleration : Inport
  velocity : Inport  Port=2
  position : Inport  Port=3
  Complementary Filter : mspfiltlib/Complementary Filter  DispRefFrame=NED  OrientationFormat=Rotation matrix  AccelerometerGain=0.01  HasMagnetometer=on  MagnetometerGain=0.01  SimulateUsing=Interpreted execution
  Display{3..7} (5 alike) : Display
  IMU : mspsensorlib/IMU  DispRefFrame=NED  TemperaturePort=off  Temperature=25  MagneticFieldPort=off  MagneticFieldNED=[ 27.5550, -2.4169, -16.0849 ]  MagneticFieldENU=[ -2.4169, 27.5550, 16.0849 ]  SeedDouble=67  SimulateUsing=Interpreted execution  AccelParamsMeasurementRange=Inf  AccelParamsResolution=0  AccelParamsConstantBias=[ 0, 0, 0 ]  AccelParamsAxesMisalignment=[ 100, 0, 0; 0, 100, 0; 0, 0, 100 ]  AccelParamsNoiseDensity=[ 0, 0, 0 ]  AccelParamsBiasInstability=[ 0, 0, 0 ]  AccelParamsBiasInstabilityNumerator=fractalcoef().Numerator  AccelParamsBiasInstabilityDenominator=fractalcoef().Denominator  AccelParamsRandomWalk=[ 0, 0, 0 ]  AccelParamsNoiseType=double-sided  AccelParamsTemperatureBias=[ 0, 0, 0 ]  AccelParamsTemperatureScaleFactor=[ 0, 0, 0 ]  GyroParamsMeasurementRange=Inf  GyroParamsResolution=0  GyroParamsConstantBias=[ 0, 0, 0 ]  GyroParamsAxesMisalignment=[ 100, 0, 0; 0, 100, 0; 0, 0, 100 ]  GyroParamsAccelerationBias=[ 0, 0, 0 ]  GyroParamsNoiseDensity=[ 0, 0, 0 ]  GyroParamsBiasInstability=[ 0, 0, 0 ]  GyroParamsBiasInstabilityNumerator=fractalcoef().Numerator  GyroParamsBiasInstabilityDenominator=fractalcoef().Denominator  GyroParamsRandomWalk=[ 0, 0, 0 ]  GyroParamsNoiseType=double-sided  GyroParamsTemperatureBias=[ 0, 0, 0 ]  GyroParamsTemperatureScaleFactor=[ 0, 0, 0 ]  MagParamsMeasurementRange=Inf  MagParamsResolution=0  MagParamsConstantBias=[ 0, 0, 0 ]  MagParamsAxesMisalignment=[ 100, 0, 0; 0, 100, 0; 0, 0, 100 ]  MagParamsNoiseDensity=[ 0, 0, 0 ]  MagParamsBiasInstability=[ 0, 0, 0 ]  MagParamsBiasInstabilityNumerator=fractalcoef().Numerator  MagParamsBiasInstabilityDenominator=fractalcoef().Denominator  MagParamsRandomWalk=[ 0, 0, 0 ]  MagParamsNoiseType=double-sided  MagParamsTemperatureBias=[ 0, 0, 0 ]  MagParamsTemperatureScaleFactor=[ 0, 0, 0 ]
  MATLAB Function : MATLAB Function  TreatAsAtomicUnit=on
  MATLAB Function1 : MATLAB Function  TreatAsAtomicUnit=on
  MATLAB Function2 : MATLAB Function  TreatAsAtomicUnit=on
  Selector : Selector  InputPortWidth=6  IndexOptions=Index vector (dialog)  Indices=[1 2 3]  OutputSizes=1
  Selector1 : Selector  InputPortWidth=6  IndexOptions=Index vector (dialog)  Indices=[4 5 6]  OutputSizes=1
  Zero-Order Hold : ZeroOrderHold  SampleTime=-1
  Zero-Order Hold1 : ZeroOrderHold  SampleTime=-1
  Zero-Order Hold2 : ZeroOrderHold  SampleTime=-1
  wires:
  IMU/2 -> Display6/1, Complementary Filter/2
  Complementary Filter/1 -> Display3/1
  IMU/3 -> Display7/1, Complementary Filter/3
  IMU/1 -> Display5/1, Complementary Filter/1
  Selector/1 -> MATLAB Function1/1(x)
  Selector1/1 -> MATLAB Function2/1(x)
  Zero-Order Hold/1 -> IMU/1
  MATLAB Function1/1(y) -> Zero-Order Hold/1
  Complementary Filter/2 -> Display4/1
  MATLAB Function/1(R) -> Zero-Order Hold2/1
  Zero-Order Hold2/1 -> IMU/3
  Zero-Order Hold1/1 -> IMU/2
  velocity/1 -> Selector1/1
  MATLAB Function2/1(y) -> Zero-Order Hold1/1
  Acceleration/1 -> Selector/1
  position/1 -> MATLAB Function/1(eul)

== system dart_AUV_simulink_model/ 6DoF Dynamic Equations /Inverse Mass Matrix ==
  Thrust force : Inport
  inv(Total Mass) : Gain  Gain=inv(Mt)  Multiplication=Matrix(K*u)  OutDataTypeStr=Inherit: Same as input  ParamDataTypeStr=Inherit: Same as input
  Acceleration : Outport  VectorParamsAs1DForOutWhenUnconnected=off
  wires:
  inv(Total Mass)/1 -> Acceleration/1
  Thrust force/1 -> inv(Total Mass)/1

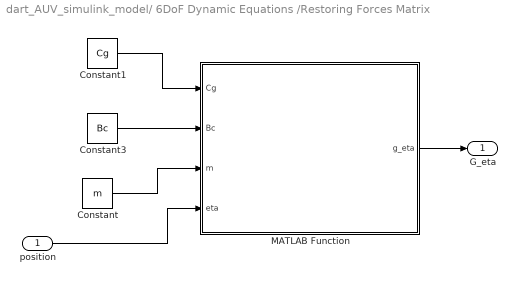
== system dart_AUV_simulink_model/ 6DoF Dynamic Equations /Restoring Forces Matrix ==
  position : Inport
  Constant : Constant  Value=m
  Constant1 : Constant  Value=Cg
  Constant3 : Constant  Value=Bc
  MATLAB Function : MATLAB Function  TreatAsAtomicUnit=on
  G_eta : Outport
  wires:
  position/1 -> MATLAB Function/4(eta)
  Constant/1 -> MATLAB Function/3(m)
  Constant1/1 -> MATLAB Function/1(Cg)
  Constant3/1 -> MATLAB Function/2(Bc)
  MATLAB Function/1(g_eta) -> G_eta/1

== matlab function dart_AUV_simulink_model/ 6DoF Dynamic Equations /Restoring Forces Matrix/MATLAB Function ==
  data: Cg input; Bc input; m input; eta input; g_eta output

function g_eta = g_eta_fun(Cg, Bc,m, eta)
    zg = Cg(3);
    zb = Bc(3);
    g = 9.81;
    BGz = zb-zg;
    phi   = eta(4);
    theta = eta(5);
    W = m * g;
    B = 2.25 * g;
    g_eta = [ (W - B) * sin(theta);
             -(W - B) * cos(theta) * sin(phi);
             -(W - B) * cos(theta) * cos(phi);
              BGz*W*cos(theta)*sin(phi);
              BGz*W*sin(theta);
              0
             ];
end

== matlab function dart_AUV_simulink_model/ 6DoF Dynamic Equations /Centripetal and Coriolis Matrices /MATLAB Function ==
  data: v input; CRB output; m input; Cg input; I input; Ma input; CA output
function [CRB, CA] = CoriolisMatrices(v, m, Cg, I, Ma)
    % Moments of Inertia
    Ixx = I(1); Iyy = I(2); Izz = I(3);
    
    % Linear and Angular Velocities
    v_lin = v(1:3);  % [u, v, w]
    v_ang = v(4:6);  % [p, q, r]

    % Skew-Symmetric Matrix Function
    S = @(x) [  0   -x(3)  x(2);
               x(3)   0   -x(1);
              -x(2)  x(1)   0];

    % Rigid-Body Coriolis Matrix (CRB)
    CRB = [
        zeros(3,3), S(m * v_lin + m * cross(v_ang, Cg));
        S(m * v_lin + m * cross(v_ang, Cg)), S([Ixx; Iyy; Izz] .* v_ang)
    ];

    % Added Mass Coriolis Matrix (CA)
    F1 = Ma(1:3,1:3) * v_lin + Ma(1:3,4:6) * v_ang;
    F2 = Ma(4:6,1:3) * v_lin + Ma(4:6,4:6) * v_ang;

    CA = [ zeros(3,3), -S(F1);
           -S(F1),     -S(F2) ];

end

== matlab function dart_AUV_simulink_model/ 6DoF Dynamic Equations / A Matrix/MATLAB Function ==
  data: data input; u input; y output
function y = fcn(data, u)

y = zeros(6,1);
y =[0 -u(6) u(5) 0 0 0;u(6) 0 -u(4) 0 0 0;-u(5) u(4) 0 0 0 0;0 0 0 0 0 0;0 0 0 0 0 0;0 0 0 0 0 0]*data;

== matlab function dart_AUV_simulink_model/ 6DoF Dynamic Equations /Hydrodynamic Damping Matrices /MATLAB Function ==
  data: CD input; CL input; DL output; rho input; R input; L input; DNL output
function [DL, DNL] = computeDampingMatrices(CD,CL, rho, R, L)
    % Computes Linear and Quadratic Damping Matrices for an AUV.
    %
    % Inputs:
    %   CD    - Drag coefficients [Xu, Yv, Zw, Kp, Mq, Nr] (1x6)
    %   CL    - Lift Coefficients [Kpp, Mqq, Nrr]
    %   rho   - Water density (kg/m^3)
    %   R     - AUV radius (m)
    %   L     - Characteristic length (e.g., fin span, m)
    %   alpha - Empirical scaling factor for linear damping (0.1 to 0.3)
    %
    % Outputs:
    %   DL  - Linear damping matrix (6x6)
    %   DNL - Quadratic damping matrix (6x6)

    % Compute Cross-sectional Area
    A = pi * R^2; % (m^2)

    % Compute Quadratic Damping Coefficients (DNL)
    % Xu_nl = 0.5 * rho * A * CD(1); % Surge
    % Yv_nl = 0.5 * rho * A * CD(2); % Sway
    % Zw_nl = 0.5 * rho * A * CD(3); % Heave
    % Kp_nl = 0.5 * rho * A * L * CL(1); % Roll
    % Mq_nl = 0.5 * rho * A * L * CL(2); % Pitch
    % Nr_nl = 0.5 * rho * A * L * CL(3); % Yaw
        % Compute Quadratic Damping Coefficients (DNL)
    Xu_nl = 0.5 * rho * A * CD(1); % Surge
    Yv_nl = 0.5 * rho * A * CD(2); % Sway
    Zw_nl = 0.5 * rho * A * CD(3); % Heave
    Kp_nl = 0.5 * rho * A * L * CL(1); % Roll
    Mq_nl = 0.5 * rho * A * L * CL(2); % Pitch
    Nr_nl = 0.5 * rho * A * L * CL(3); % Yaw
    % Construct Quadratic Damping Matrix
    DNL = diag([Xu_nl, 0, 0, 0, 0, 0; 
                0, Yv_nl, 0, 0, 0, 0; 
                0, 0, Zw_nl, 0, 0, 0; 
                0, 0, 0, Kp_nl, 0, 0; 
                0, 0, 0, 0, Mq_nl, 0; 
                0, 0, 0, 0, 0, Nr_nl]);
    alpha = 0.2;
    % Compute Linear Damping Coefficients (DL) as a fraction of DNL
    Xu = alpha * Xu_nl; % Surge
    Yv = alpha * Yv_nl; % Sway
    Zw = alpha * Zw_nl; % Heave
    Kp = alpha * Kp_nl; % Roll
    Mq = alpha * Mq_nl; % Pitch
    Nr = alpha * Nr_nl; % Yaw

    % Construct Linear Damping Matrix
    DL = diag([Xu, 0, 0, 0, 0, 0; 
               0, Yv, 0, 0, 0, 0; 
               0, 0, Zw, 0, 0, 0; 
               0, 0, 0, Kp, 0, 0; 
               0, 0, 0, 0, Mq, 0; 
               0, 0, 0, 0, 0, Nr]);

end

== matlab function dart_AUV_simulink_model/ 6DoF Dynamic Equations /IMU with Filtering/MATLAB Function ==
  data: eul input; R output
function R = eul2R(eul)

% Extract [roll, pitch, yaw] from eul = [x y z roll pitch yaw]
angles = eul(4:6);  % This will be a 1x3 or 3x1

% Reshape to 1x3 row vector 
angles = reshape(angles, 1, 3);

% rotation matrix
R = eul2rotm(angles, 'XYZ');
end

== matlab function dart_AUV_simulink_model/ 6DoF Dynamic Equations /IMU with Filtering/MATLAB Function1 ==
  data: x input; y output
function y = toRow(x)

y = reshape(x, 1, []);

== matlab function dart_AUV_simulink_model/ 6DoF Dynamic Equations /IMU with Filtering/MATLAB Function2 ==
  data: x input; y output
function y = toRow(x)

y = reshape(x, 1, []);

== matlab function dart_AUV_simulink_model/MATLAB Function ==
  data: t input; z_target output
function z_target = depth_sequence_controller(t)
% This function outputs a target depth based on simulation time.
% Sequence: Dive to 0.5m → wait 30s → dive to 1.0m → wait → dive to 1.5m → wait → return to 0m

% Define depth setpoints (in meters, negative for underwater)
depths = [0.5, 1.0, 1.5, 0.0];

% Wait duration at each depth (in seconds)
wait_time = 30;

% Total duration per stage (including wait)
stage_duration = wait_time;

% Calculate the current stage based on time
stage = floor(t / stage_duration) + 1;

% Limit the stage index to the available number of depths
if stage <= length(depths)
    z_target = -depths(stage); % Convert to negative for depth
else
    z_target = -depths(end); % Stay at final depth
end

end

== matlab function dart_AUV_simulink_model/Thruster Model/MATLAB Function ==
  data: F input; P output
function P = thrust_power(F)
% Continuous power cost function for APISQUENN U2 thruster
% Input:
%   F - Thrust force in Newtons (can be scalar or vector)
% Output:
%   P - Power in Watts (same shape as F)

% Convert Newtons to kg-equivalent
F_kg = F;

% Voltage
V = 16;

% Preallocate output
P = zeros(size(F_kg));

% Polynomial coefficients 
% Forward: I = a_f * T + b_f
a_f = 5.0;
b_f = -0.5;

% Reverse: I = a_r * T + b_r
a_r = -5.0;
b_r = -0.5;

% Compute current and power for each element
for i = 1:length(F_kg)
    T = F_kg(i);
    
    % Clamp T to valid range
    T = max(min(T, 1.7), -1.6);

    if T >= 0
        I = a_f * T + b_f;
    else
        I = a_r * T + b_r;
    end

    
    I = max(I, 0);  % Power can’t be negative

    % Compute power
    P(i) = V * I;
end
end

== matlab function dart_AUV_simulink_model/Current /NED to Body Frame1 ==
  data: eta input; y output; u input
function y = rotation_matrix(eta,    u)
  
  % eta = wrapToPi(eta(3));

  rot_eta = [cos(eta(3)) -sin(eta(3)) 0;
             sin(eta(3)) cos(eta(3)) 0;
             0 0 1];

  % u(3) = wrapToPi(u(3));

  %rot_eta = rotz(eta(3));
  p_comp = rot_eta.' * u;


y = p_comp;
